simulink model "nnc"  (R2014a)
settings: Solver=VariableStepAuto  StartTime=0.0  StopTime=120  RelTol=1e-3  AbsTol=1e-6
undefined symbols (not defined in the file): now, sfunxy2
settings Model: ExtModeTrigMode=oneshot  ExtModeArmWhenConnect=off  TunableVars=prueba  TunableVarsStorageClass=Auto  Creator=The MathWorks, Inc.  LastModifiedBy=Administrator
settings DataIOCC: LimitDataPoints=off  SaveOutput=off  SignalLoggingName=sigsOut
settings OptimizationCC: BooleanDataType=off  DefaultParameterBehavior=Inlined  ExpressionDepthLimit=2147483647  InitFltsAndDblsToZero=on  SimCompilerOptimization=off
settings DebuggingCC: SaveWithParameterizedLinksMsg=none  UnderspecifiedInitializationDetection=Classic  SignalResolutionControl=TryResolveAllWithWarning  SolverPrmCheckMsg=none  MultiTaskDSMMsg=warning  MultiTaskCondExecSysMsg=none  FcnCallInpInsideContextMsg=warning  FrameProcessingCompatibilityMsg=error  StateNameClashWarn=warning  SFExecutionAtInitializationDiag=none
settings HardwareCC: ProdBitPerSizeT=32  ProdBitPerPtrDiffT=32  TargetUnknown=on
settings RTWCC: TemplateMakefile=grt_vc.tmf  RTWCompilerOptimization=off
settings GRTTargetCC: TargetFcnLib=ansi_tfl_tmw.mat  CombineOutputUpdateFcns=off  GRTInterface=on
settings ConfigComp: CovMetricSettings=dw  CovHtmlReporting=on  CovSaveCumulativeToWorkspaceVar=on  CovSaveSingleToWorkspaceVar=on  CovExternalEMLEnable=off

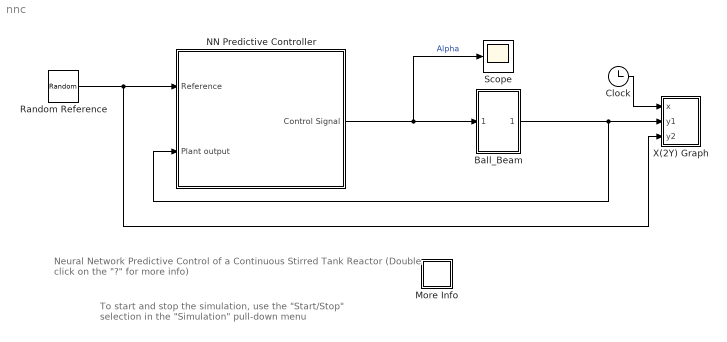
== system nnc ==
  note: Neural Network Predictive Control of a Continuous Stirred Tank Reactor
      | (Double click on the "?" for more info)
  note: To start and stop the simulation, use the "Start/Stop"
      | selection in the "Simulation" pull-down menu
  Ball_Beam : Subsystem
  Clock : Clock
  More Info : Subsystem
      mask Display: disp('?')
  NN Predictive Controller : Subsystem  mask(NN Predictive Controller){N2=30, Nu=5, Ts=0.02, rho=0.006, alpha=0.0038, csrchfun=csrchbac, maxiter=2, S1=50, Ni=2, Nj=2, sim_file=bblim, trainfun=trainlm, Use_validation=1, Use_Testing=1, max_i=1.5708, min_i=-1.5708, sam_training=6000, epochs=1000, minp=-1.5334084584548999, maxp=1.5679109681822905, mint=-0.02130316380495214, maxt=1.5679109681822905, Normalize=0, IW=[0.22491991621003873 0.0098832626431852137;-1.0076662341871958 -1.9876559909740914;0.049858716964002125 -0.053692169279735996;0.87062372932385801 0.82190537833118216;0.12344136598622515 -0.17527555943156486;0.17352805770747334 1.4765184818877881;0.23993382136993954 -0.40935491975370436;-0.43722309067762299 0.52692444912700132;-0.55134774376918627 0.56774514157696188;0.47948521878792216 0.82881036914491113;1.4771748889751788 1.4353693252018802;-1.4042679387847912 -0.71944601597907065;-1.211446940550243 -0.56926402765455519;0.5477219424090588 -0.91352178528008054;0.39676796380956808 1.5088925623991185;-0.0037467591273643405 0.0047439140681983785;0.15005208752012419 -0.23650360552910485;1.4027621065498275 -1.1331145434270191;-0.81650546524969991 -0.28357460087503983;-1.2440567403914755 -1.6375261708134348;-1.8518838271368887 0.63789785170132585;-1.0658218071751555 -0.36299584192834483;0.3208165341093539 -0.58827405586371107;0.57957905764975692 -0.96659200969995196;-1.3221151575616512 0.91670981738763258;0.92386347091713183 0.54309097628481007;0.71360769364797505 -0.27665373901699175;0.61781933146853907 1.9105705099458092;-1.4899145482971261 -1.378536397255133;0.52170509180144908 0.81455623333773519;0.085713436101469406 -0.11005735027508509;1.0903741057425522 0.24024988174866127;1.018688765237562 -1.042685594645091;1.0552667986195889 0.50534552475525962;0.13320292710658455 -0.21524507394952513;-0.18407967764866251 -1.023870635850014;-0.37933027499603117 -0.75351817518537201;-1.7038298644322791 1.7995530185582662;-0.0014896724185785165 -0.00044902663204694489;1.6303459273884244 -0.81055228351810737;-0.76510180650824222 -1.8730482977765301;-1.3446258578008321 -0.47271911292904539;-0.3998247134414688 -1.5748541591431509;-0.14120515690113095 0.24342259870860067;0.34894654455003604 -0.38657115707644812;-1.7019499153237525 -0.71515563985607367;1.6714063260699963 -0.29428644475821891;-0.089837106315165741 0.091873318942910939;1.1095709751334788 -0.9362805750595895;-0.1387717799400161 0.21718410483985612], LW1_2=[4.4623327463656812 4.1315658841457683;-0.94388621690037411 1.1846755419084363;-5.3135762131563622 2.9306343898983886;-3.0748301772054463 5.4843159863178794;-0.91437537143530223 7.0182481206312772;-2.5888858858570258 -5.5458706199150836;-2.836651610943441 5.1310548126469344;3.4731480884742592 1.0848990215988317;-1.2124507653280949 7.1246400279307469;5.0090014089234494 0.2677270525311618;-1.2249385873643528 -0.20144613867092209;4.117706908095089 4.6677669592722593;-1.6027523387141496 -4.6422722145507871;7.0934271855639848 -0.18744657698215611;3.3699954108751977 5.0432581202323545;-1.7187768300315172 0.84875621705096438;-3.6669391771378539 3.2291614548906025;3.2023094523125493 2.5108890318796981;5.230388086700529 1.2417420096782938;-1.625546211219437 -2.4675776777109322;3.0478625246308546 2.8934194367998569;-0.31541093459694725 -5.5945525047621869;4.7676564460638771 1.0626760104197048;4.5859698311121981 2.6336953872700386;-3.6265459579291854 2.316692776935811;3.3356488704913212 3.3904226676864861;4.7329997132498178 4.6599226047025306;0.49224071693750993 3.7623541153780025;3.9315311901854653 0.73334486421216605;0.24528836960714684 5.0047647593570019;-3.3094466286757869 1.7525276793521691;-2.7950037402956514 -4.8715063657360806;-1.0523925214006713 -4.3247522130262794;3.5078107249679267 5.2839067802350321;5.9032372575841814 -1.4557021531682095;2.9358708796561115 3.6695512465895299;-2.3284344121646749 -3.2497495961191563;0.29850678735929026 0.51857317631551814;-2.6219983593383662 1.3327193073085353;-3.4129598855462056 -4.3758486641729961;-4.5554505635706555 1.1124837452050258;4.0902385201642435 -3.569358868514017;-0.41346661090285186 -4.9729836740265592;-3.148354526037517 0.76924601955381422;-0.4844867888029139 -4.983579813505024;-3.1802773483702413 -3.5837917778157746;-4.8631372802657724 -3.1700172807335218;5.6639502736372025 -4.7686746750111801;0.42353984400092332 -3.9548404538917676;4.5103020318933531 -3.7284796187834126], LW2_1=[0.00051946813025846941 -3.3442905937980359e-06 -0.30860798511542337 -1.5468962392643881e-05 -0.00082636716886553489 -2.1013219881474448e-05 0.064236929100461915 0.0010137732852358299 0.00048575415620022997 7.0410210338688942e-05 -1.3897061033928293e-06 1.248176705416512e-06 4.0185284080181121e-05 6.1050770024674008e-05 9.2921792788198899e-06 -0.96460792204542134 -0.0080751512784448254 4.2110888956642545e-05 4.0498328292793391e-08 8.2679926606762124e-07 9.9221966581924357e-06 5.4683248878955386e-05 0.0012303225316798753 -0.00042267890935354625 -3.9036754602669728e-05 5.4586215727336794e-05 2.6527545457523084e-05 -1.2024500517166156e-06 3.0923755319074621e-06 -6.022751697421131e-06 -0.034939523943512261 -4.2902615867908329e-08 6.5765306392467731e-05 1.2343196433984512e-07 0.0022613200374336888 1.9611281895911073e-05 -2.1427493931934968e-05 2.2225513391004542e-05 -0.47070200078283703 -3.1445263989671769e-06 -1.3653933784670748e-05 9.596257304070624e-06 -2.6196983497115524e-07 -0.0081311597557210992 -0.0026278006826996997 3.4264009712070663e-06 -2.4476978420323782e-08 0.66735755107770778 -0.00022533058869324954 0.59818146811133466], B1=[-8.6067221197490706;3.2459652847270819;4.4104273528387266;0.75583018532547563;0.080816605439676392;6.8203560574108346;2.9889071463929189;-4.012091397415344;-0.91363166110731175;-4.4488832882852281;3.1915208862697035;-5.8870867269930267;5.2266436095632098;-4.7478458387830829;-5.892706965164102;0.87070304834985146;1.1366135810675007;-4.0844048909348611;-3.8502563212011989;3.4321879961878929;-3.6537610024035123;3.2251693809792958;-3.1805778591858025;-3.9669209371014449;0.73341742754796324;-3.5708604255432612;-4.999266660144837;-2.1041385010514069;-2.115512526933335;-1.9443825965313872;0.66369474845259357;3.034873653124357;1.4373104805754686;-3.0693195350912199;-1.4863852874596262;-1.3567515627524569;1.8939052560517329;0.62217518869239818;-0.43738143974634336;2.1320843253251307;-0.85744005694978243;1.8204149649629238;-0.18109927751243141;-0.12626191214293536;-0.54342626113892878;0.16684812743323538;0.6431049801975669;3.5344635286735455;5.1703776800916081;4.0524421048987485], B2=-0.50647878860674611, max_i_int=1, min_i_int=0.02, limit_output=1, max_output=1, min_output=0, Use_Previous_Weights=1}
      mask prompts: Ts "Sample time"; rho "rho (typically = 0.03)"; alpha "alpha (typically = 0.001)"; csrchfun "Minimization rutine"; trainfun "Training function"
      mask help: NN Predictive Controller. You first train a neural network model of the plant to be controlled. The controller uses the plant model to predict plant performance over a specified time horizon. An optimization algorithm determines the control signal that optimizes plant performance over this horizon. Double click the NN Predictive Controller block to train the plant model and set the controller parameters.
      mask init:
      | xl = [0   .53   .53     .85   .85  .53  .53  NaN .85  .92 .92];
      | yl = [.95 .95 1.05  1.05   .82  .82  .95  NaN  .95 .95 .65];
      | x2 = [0 .53    NaN .92 1.2 NaN .53 .85 .85 .53 .53 ];
      | y2 = [.39 .39   NaN .65 .65 NaN .59 .59 .29 .29  .59];
      | x3 = [.67 .67 NaN .64 .67 .70 NaN .53 .4   .4   .53 NaN .46 .53 .46];
      | y3 = [.59 .82 NaN .66 .59 .66 NaN .55 .55 .86 .86 NaN  .89 .86 .83];
      | 
      | x1t=.03; y1t=.31;
      | x2t=.03; y2t=.8;
      | x8t=.03;y8t=.21;
      | x3t=.77; y3t=.53;
      | x4t=.77; y4t=.44;
      | x5t=.45; y5t=.76;
      | x6t=.45; y6t=.35;
      | x7t=.45; y7t=.25;
      settings: OpenFcn=nncontrolutil('nnpredict','',gcbh,gcb);
      mask TypeOptions csrchfun: csrchgol | csrchbac | csrchhyb | csrchbre | csrchcha
      mask TypeOptions trainfun: trainbfg | trainbr  | traincgb | traincgf | traincgp | traingd | traingdm | traingda | traingdx | trainlm  | trainoss | trainrp  | trainscg
      mask Display:
      | plot([[xl NaN x2]*.9-.075 ], [[yl  NaN y2]*.9-.1 ]);
      | plot([[x3]*.9-.075 ], [[y3]*.9-.1 ]);
      | text(x1t,y1t,'Plant');
      | text(x8t,y8t,'Output');
      | text(x2t,y2t,'Reference');
      | text(x3t,y3t,'Control');
      | text(x4t,y4t,'Signal');
      | text(x5t,y5t,'Optim.');
      | text(x6t,y6t,'NN');
      | text(x7t,y7t,'Model');
  Random Reference : UniformRandomNumber  Minimum=0  Maximum=0.4  Seed=round(now)  SampleTime=6
  Scope : Scope
  X(2Y) Graph : Subsystem  LoadFcn=sfunxy2([],[],[],'LoadBlock')  StartFcn=sfunxy2([],[],[],'Start')  StopFcn=sfunxy2([],[],[],'Stop')  mask(X(2Y) scope.){xmin=0, xmax=1, ymin=0, ymax=0.5, st=-1}
      mask prompts: xmin "x-min:"; xmax "x-max:"; ymin "y-min:"; ymax "y-max:"; st "Sample time:"
      mask help: X(2Y) scope using MATLAB graph window. First input is used as time base. Enter plotting ranges.
      settings: CopyFcn=sfunxy2([],[],[],'CopyBlock')  DeleteFcn=sfunxy2([],[],[],'DeleteBlock')  NameChangeFcn=sfunxy2([],[],[],'NameChange')
      mask Help: This block can be used to explore limit cycles. Look at function sfunxy.m to see how it works.
      mask Display: plot([.05 .95 .95 .05 .05],[.45 .45 .95 .95 .45], 0.5+cos(0:0.1:2*pi)*0.3,0.7+sin(0:0.1:2*pi)*0.2)
  wires:
  Clock/1 -> X(2Y) Graph/1(x)
  NN Predictive Controller/1(Control Signal) -> Ball_Beam/1(In1), Scope/1  "Alpha"
  Random Reference/1 -> NN Predictive Controller/1(Reference), X(2Y) Graph/3(y2)
  Ball_Beam/1(Out1) -> X(2Y) Graph/2(y1), NN Predictive Controller/2(Plant output)

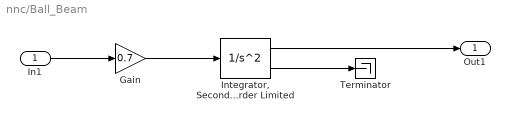
== system nnc/Ball_Beam ==
  In1 : Inport
  Gain : Gain  Gain=0.7
  "Integrator, Second-Order Limited" : SecondOrderIntegrator  LimitX=on  UpperLimitX=0.4  LowerLimitX=0  LimitDXDT=on
  Terminator : Terminator
  Out1 : Outport
  wires:
  In1/1 -> Gain/1
  "Integrator, Second-Order Limited"/1 -> Out1/1
  Gain/1 -> "Integrator, Second-Order Limited"/1
  "Integrator, Second-Order Limited"/2 -> Terminator/1

== system nnc/More Info ==
  note: This system simulates predictive control
      | of a continuous stirred tank reactor.
  note: Double-click on the NN Predictive Controller block
      | to set the controller parameters and train the plant model.
  note: For more information on what the controller
      | does, look under the mask of the NN Predictive
      | Controller block and look at the S-function p_opt2.m.

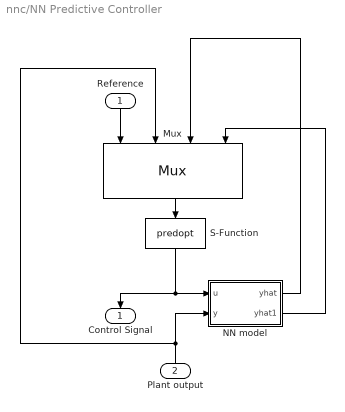
== system nnc/NN Predictive Controller ==
  Reference : Inport
  Plant output : Inport  Port=2
  Mux : Mux
      settings: DisplayOption=signals
  NN model : Subsystem
  S-Function : S-Function  FunctionName=predopt  Parameters=N2,Ts,Nu,maxiter,csrchfun,rho,alpha,S1,IW,LW1_2,LW2_1,B1,B2,Ni,Nj,min_i,max_i,minp,maxp,mint,maxt,Normalize  EnableBusSupport=off
  Control Signal : Outport
  wires:
  Mux/1 -> S-Function/1
  S-Function/1 -> NN model/1(u), Control Signal/1
  NN model/2(yhat1) -> Mux/4
  NN model/1(yhat) -> Mux/3
  Reference/1 -> Mux/1
  Plant output/1 -> NN model/2(y), Mux/2

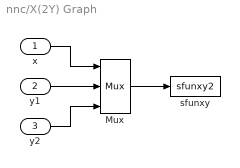
== system nnc/X(2Y) Graph ==
  x : Inport
  y1 : Inport  Port=2
  y2 : Inport  Port=3
  Mux : Mux  Inputs=3
  sfunxy : S-Function  FunctionName=sfunxy2  Parameters=[xmin xmax ymin ymax], st  EnableBusSupport=off
  wires:
  y2/1 -> Mux/3
  y1/1 -> Mux/2
  x/1 -> Mux/1
  Mux/1 -> sfunxy/1

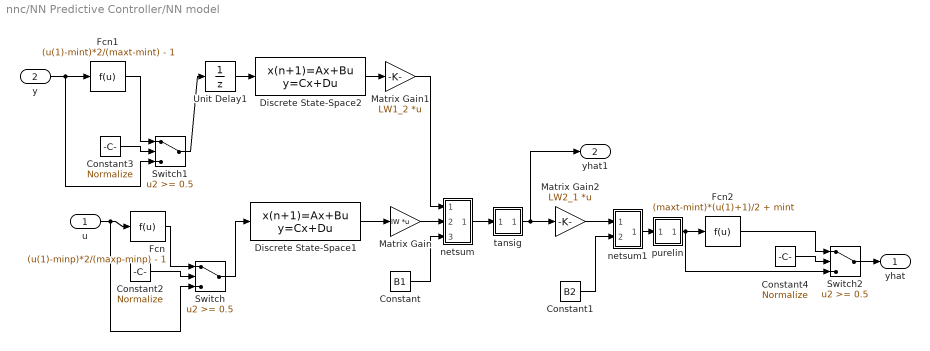
== system nnc/NN Predictive Controller/NN model ==
  u : Inport
  y : Inport  Port=2
  Constant : Constant  Value=B1
  Constant1 : Constant  Value=B2
  Constant2 : Constant  Value=Normalize
  Constant3 : Constant  Value=Normalize
  Constant4 : Constant  Value=Normalize
  Discrete State-Space1 : DiscreteStateSpace  A=[0 zeros(1,Ni-2);eye(Ni-2,Ni-1)]  B=[zeros(double(Ni==1));eye(Ni-1,1)]  C=[0 zeros(1,Ni-2);eye(Ni-1,Ni-1)]  D=eye(Ni,1)  SampleTime=Ts
  Discrete State-Space2 : DiscreteStateSpace  A=[0 zeros(1,Nj-2);eye(Nj-2,Nj-1)]  B=[zeros(double(Nj==1));eye(Nj-1,1)]  C=[0 zeros(1,Nj-2);eye(Nj-1,Nj-1)]  D=eye(Nj,1)  SampleTime=Ts
  Fcn : Fcn  Expr=(u(1)-minp)*2/(maxp-minp) - 1
  Fcn1 : Fcn  Expr=(u(1)-mint)*2/(maxt-mint) - 1
  Fcn2 : Fcn  Expr=(maxt-mint)*(u(1)+1)/2 + mint
  Matrix Gain : Gain  Gain=IW  Multiplication=Matrix(K*u)  SaturateOnIntegerOverflow=on  OutDataTypeStr=Inherit: Same as input  ParamDataTypeStr=Inherit: Same as input
  Matrix Gain1 : Gain  Gain=LW1_2  Multiplication=Matrix(K*u)  SaturateOnIntegerOverflow=on  OutDataTypeStr=Inherit: Same as input  ParamDataTypeStr=Inherit: Same as input
  Matrix Gain2 : Gain  Gain=LW2_1  Multiplication=Matrix(K*u)  SaturateOnIntegerOverflow=on  OutDataTypeStr=Inherit: Same as input  ParamDataTypeStr=Inherit: Same as input
  Switch : Switch  Threshold=0.5  ZeroCross=off  SaturateOnIntegerOverflow=on  InputSameDT=on
  Switch1 : Switch  Threshold=0.5  ZeroCross=off  SaturateOnIntegerOverflow=on  InputSameDT=on
  Switch2 : Switch  Threshold=0.5  ZeroCross=off  SaturateOnIntegerOverflow=on  InputSameDT=on
  Unit Delay1 : UnitDelay  SampleTime=Ts
  netsum : Subsystem
      mask Display: disp('+')
  netsum1 : Subsystem
      mask Display: disp('+')
  purelin : Subsystem
      mask Display: plot([-1 1],[0 0],[-1 1],[-1 1])
  tansig : Subsystem
      mask Display: plot([-1 1],[0 0],[-1 -.9 -.8 -.7 -.6 -.5 -.4 -.3 -.2 -.1 0 .1 .2 .3 .4 .5 .6 .7 .8 .9 1],2./(1+exp(-8*[-1 -.9 -.8 -.7 -.6 -.5 -.4 -.3 -.2 -.1 0 .1 .2 .3 .4 .5 .6 .7 .8 .9 1]))-1)
  yhat : Outport
  yhat1 : Outport  Port=2
  wires:
  netsum1/1(Out1) -> purelin/1(n)
  Constant1/1 -> netsum1/2(In2)
  Matrix Gain2/1 -> netsum1/1(In1)
  netsum/1(Out1) -> tansig/1(n)
  Constant/1 -> netsum/3(In3)
  Matrix Gain1/1 -> netsum/1(In1)
  Matrix Gain/1 -> netsum/2(In2)
  tansig/1(a) -> Matrix Gain2/1, yhat1/1
  Discrete State-Space1/1 -> Matrix Gain/1
  Fcn/1 -> Switch/1
  Switch/1 -> Discrete State-Space1/1
  u/1 -> Fcn/1, Switch/3
  Constant2/1 -> Switch/2
  Discrete State-Space2/1 -> Matrix Gain1/1
  Unit Delay1/1 -> Discrete State-Space2/1
  Constant3/1 -> Switch1/2
  Switch1/1 -> Unit Delay1/1
  Fcn1/1 -> Switch1/1
  y/1 -> Fcn1/1, Switch1/3
  Constant4/1 -> Switch2/2
  Switch2/1 -> yhat/1
  Fcn2/1 -> Switch2/1
  purelin/1(a) -> Fcn2/1, Switch2/3

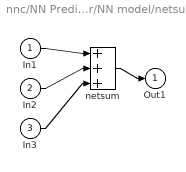
== system nnc/NN Predictive Controller/NN model/netsum ==
  In1 : Inport
  In2 : Inport  Port=2
  In3 : Inport  Port=3
  netsum : Sum  Inputs=3  SaturateOnIntegerOverflow=on  InputSameDT=on  OutDataTypeStr=Inherit: Same as first input
  Out1 : Outport
  wires:
  In1/1 -> netsum/1
  In2/1 -> netsum/2
  In3/1 -> netsum/3
  netsum/1 -> Out1/1

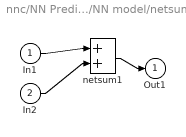
== system nnc/NN Predictive Controller/NN model/netsum1 ==
  In1 : Inport
  In2 : Inport  Port=2
  netsum1 : Sum  Inputs=2  SaturateOnIntegerOverflow=on  InputSameDT=on  OutDataTypeStr=Inherit: Same as first input
  Out1 : Outport
  wires:
  In1/1 -> netsum1/1
  In2/1 -> netsum1/2
  netsum1/1 -> Out1/1

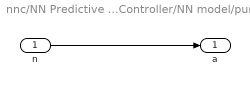
== system nnc/NN Predictive Controller/NN model/purelin ==
  n : Inport
  a : Outport
  wires:
  n/1 -> a/1

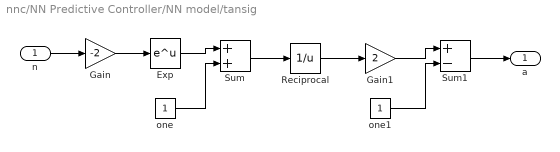
== system nnc/NN Predictive Controller/NN model/tansig ==
  n : Inport
  Exp : Math  SaturateOnIntegerOverflow=on
  Gain : Gain  Gain=-2  SaturateOnIntegerOverflow=on  OutDataTypeStr=Inherit: Same as input  ParamDataTypeStr=Inherit: Same as input
  Gain1 : Gain  Gain=2  SaturateOnIntegerOverflow=on  OutDataTypeStr=Inherit: Same as input  ParamDataTypeStr=Inherit: Same as input
  Reciprocal : Math  Operator=reciprocal  SaturateOnIntegerOverflow=on
  Sum : Sum  SaturateOnIntegerOverflow=on  InputSameDT=on  OutDataTypeStr=Inherit: Same as first input
  Sum1 : Sum  Inputs=+-  SaturateOnIntegerOverflow=on  InputSameDT=on  OutDataTypeStr=Inherit: Same as first input
  one : Constant
  one1 : Constant
  a : Outport
  wires:
  n/1 -> Gain/1
  Gain/1 -> Exp/1
  Exp/1 -> Sum/1
  one/1 -> Sum/2
  Sum/1 -> Reciprocal/1
  Reciprocal/1 -> Gain1/1
  Gain1/1 -> Sum1/1
  one1/1 -> Sum1/2
  Sum1/1 -> a/1
